simulink model "jitter"  (Simulink 2.20)
settings: Solver=ode45  StartTime=0.0  StopTime=1e-3  RelTol=1e-3  AbsTol=1e-6
undefined symbols (not defined in the file): clock, delta
settings Model: ConsistencyChecking=off  RTWPlaceOutputsASAP=off

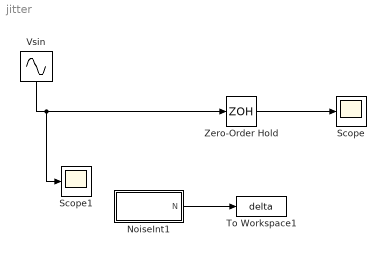
== system jitter ==
  NoiseInt1 : Subsystem
  Scope : Scope
      settings: TickLabels=on  TimeRange=auto  YMin=-5  YMax=5  SaveToWorkspace=off  SaveName=ScopeData
  Scope1 : Scope
      settings: TickLabels=on  TimeRange=auto  YMin=-5  YMax=5  SaveToWorkspace=off  SaveName=ScopeData
  To Workspace1 : ToWorkspace  VariableName=delta  SampleTime=0
      settings: Buffer=16384*32
  Vsin : Sin  Orientation=down  Amplitude=1  Frequency=2*pi*1000  Phase=0  SampleTime=0
  Zero-Order Hold : ZeroOrderHold  SampleTime=0.1e-3+delta
  wires:
  Vsin/1 -> Zero-Order Hold/1, Scope1/1
  Zero-Order Hold/1 -> Scope/1
  NoiseInt1/1(N) -> To Workspace1/1

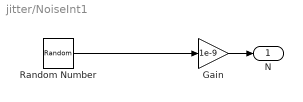
== system jitter/NoiseInt1 ==
  Gain : Gain  Gain=1e-9
  Random Number : RandomNumber  Mean=0  Variance=1  Seed=sum(clock)  SampleTime=-1
  N : Outport  Port=1  InitialOutput=0
  wires:
  Gain/1 -> N/1
  Random Number/1 -> Gain/1
